simulink model "rotpen_quick_start"  (Simulink 7.9)
settings: Solver=ode1  StartTime=0.0  StopTime=inf  FixedStep=0.002  RelTol=1e-3
PostLoadFcn:
  | qc_set_target_type(getConfigSet(bdroot, 'QUARC Default Target Configuration'));
undefined symbols (not defined in the file): HIL, qc_get_step_size
libraries: quarc_library x3, simulink_extras x2, simulink x1
settings Model: Creator=Rchan  LastModifiedBy=User  SimulationMode=external  ExtModeTrigDuration=10000  ExtModeTrigDurationFloating=10000
settings SolverCC: PositivePriorityOrder=on
settings OptimizationCC: InitFltsAndDblsToZero=on
settings DebuggingCC: SaveWithParameterizedLinksMsg=none  MultiTaskDSMMsg=warning  MultiTaskCondExecSysMsg=none  FcnCallInpInsideContextMsg=Use local settings  StrictBusMsg=None
settings RTWCC: SystemTargetFile=quarc_win64.tlc  TemplateMakefile=quarc_default_tmf  Description=QUARC Win64 Target  ProcessScript=quarc_win64_make_rtw_hook
settings STFCustomTargetCC: TargetPreCompLibLocation=C:\PROGRA~3\QUARC\lib\2012a\win64\release  CodeReplacementLibrary=ANSI_C  GeneratePreprocessorConditionals=Disable all  SystemTargetFile=quarc_win64.tlc
settings GRTTargetCC: TargetPreCompLibLocation=C:\PROGRA~3\QUARC\lib\2012a\win64\release  ParMdlRefBuildCompliant=off  CompOptLevelCompliant=off  ConcurrentExecutionCompliant=off  CombineOutputUpdateFcns=off  MatFileLogging=off  GRTInterface=on  ExtMode=on  ExtModeMexFile=quarc_comm

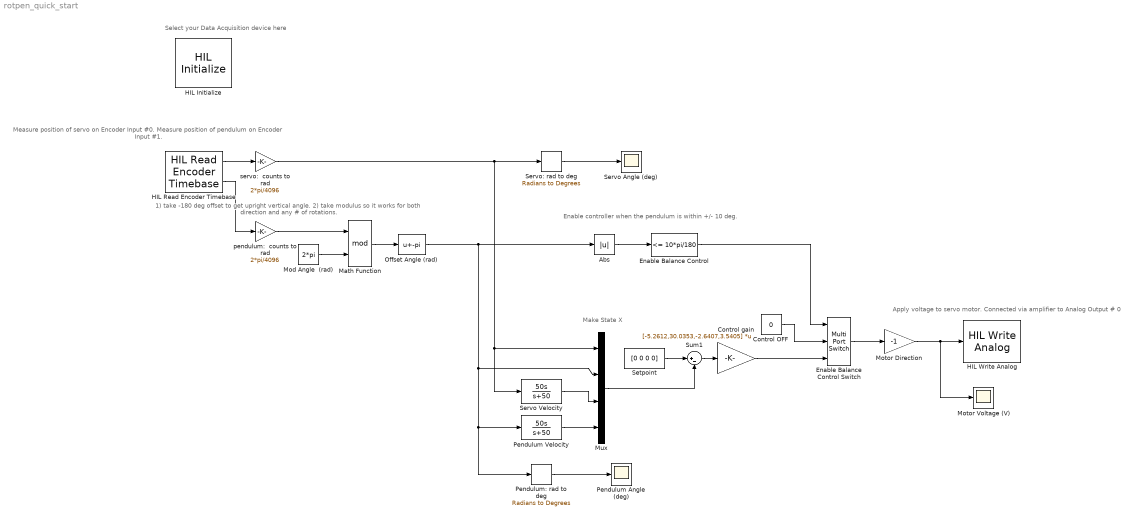
== system rotpen_quick_start ==
  note: Select your Data Acquisition device here
  note: Measure position of servo on Encoder Input #0.
      | Measure position of pendulum on Encoder Input #1.
  note: Apply voltage to servo motor.
      | Connected via amplifier to Analog Output # 0
  note: Enable controller when the
      | pendulum is within +/- 10 deg.
  note: 1) take -180 deg offset to get upright vertical angle.
      | 2) take modulus so it works for both direction
      | and any # of rotations.
  note: Make State X
  Abs : Abs
  Control OFF : Constant  Value=0
  Control gain : Gain  Gain=[-5.2612,30.0353,-2.6407,3.5405]  Multiplication=Matrix(K*u)
  Enable Balance Control : simulink/Logic and Bit Operations/Compare To Constant  relop=<=  const=10*pi/180  OutDataTypeStr=uint8  ZeroCross=off
  Enable Balance Control Switch : MultiPortSwitch  DataPortOrder=Zero-based contiguous  Inputs=2  zeroidx=on
  HIL Initialize : quarc_library/Data Acquisition/Generic/Configuration/HIL Initialize  Priority=-99  object_name=HIL-1  board_type=q8_usb  board_number=0  board_options=update_rate=normal;decimation=1  exclusive=off  active=off  hardware_clocks=[0:2]  clock_modes=[]  initial_clock_frequencies=[]  set_clock_params_at_start=off  set_clock_params_at_switch_in=off  set_clock_frequencies_at_start=off  set_clock_frequencies_at_switch_in=off  analog_input_channels=[0:7]  analog_input_maximums=10  analog_input_minimums=-10  set_analog_input_params_at_start=on  set_analog_input_params_at_switch_in=off  analog_output_channels=[0:7]  analog_output_maximums=10  analog_output_minimums=-10  initial_analog_outputs=[0]  final_analog_outputs=[0]  watchdog_analog_outputs=0  set_analog_output_params_at_start=on  set_analog_output_params_at_switch_in=off  set_analog_outputs_at_start=on  set_analog_outputs_at_switch_in=off  set_analog_outputs_at_terminate=on  set_analog_outputs_at_switch_out=off  set_analog_outputs_on_watchdog=off  digital_input_channels=[]  digital_output_channels=[]  digital_output_configuration=[]  initial_digital_outputs=[1]  final_digital_outputs=[1]  watchdog_digital_outputs=[1]  set_digital_output_params_at_start=off  set_digital_output_params_at_switch_in=off  set_digital_outputs_at_start=on  set_digital_outputs_at_switch_in=off  set_digital_outputs_at_terminate=on  set_digital_outputs_at_switch_out=off  set_digital_outputs_on_watchdog=off  encoder_channels=[0:7]  quadrature=[4]  encoder_filter_frequency=[]  initial_encoder_counts=[0]  set_encoder_params_at_start=on  set_encoder_params_at_switch_in=off  set_encoder_counts_at_start=on  set_encoder_counts_at_switch_in=off  pwm_channels=[0:7]  pwm_modes=0  pwm_frequency=99.532799999999995e6/4095  pwm_configuration=[0]  pwm_alignment=[0]  pwm_polarity=[1]  pwm_leading_deadband=[0]  pwm_trailing_deadband=[0]  initial_pwm_outputs=[0]  final_pwm_outputs=[0]  watchdog_pwm_outputs=[0]  set_pwm_params_at_start=on  set_pwm_params_at_switch_in=off  set_pwm_outputs_at_start=on  set_pwm_outputs_at_switch_in=off  set_pwm_outputs_at_terminate=on  set_pwm_outputs_at_switch_out=off  set_pwm_outputs_on_watchdog=off  other_output_channels=[]  initial_other_outputs=[]  final_other_outputs=[]  watchdog_other_outputs=[]  set_other_outputs_at_start=off  set_other_outputs_at_switch_in=off  set_other_outputs_at_terminate=off  set_other_outputs_at_switch_out=off  set_other_outputs_on_watchdog=off
  HIL Read Encoder Timebase : quarc_library/Data Acquisition/Generic/Timebases/HIL Read Encoder Timebase  object_name=HIL-1  clock=0  channels=0:1  samples_in_buffer=max(ceil(1/qc_get_step_size), 1)  active=on  vector_output=off  data_type_mode=Inherit via back propagation  data_type=double
  HIL Write Analog : quarc_library/Data Acquisition/Generic/Immediate I//O/HIL Write Analog  object_name=HIL-1  channels=0  sample_time=-1  active=off  vector_input=off
  Math Function : Math  Operator=mod  SaturateOnIntegerOverflow=on
  Mod Angle  (rad) : Constant  Value=2*pi
  "Motor Direction " : Gain  Gain=-1  SaturateOnIntegerOverflow=on  OutDataTypeStr=Inherit: Same as input  ParamDataTypeStr=Inherit: Same as input
  Motor Voltage (V) : Scope
      settings: TimeRange=10  YMin=-10  YMax=10
  Mux : Mux
  Offset Angle (rad) : Bias  Bias=-pi
  Pendulum Angle (deg) : Scope
      settings: YMin=-200  YMax=200  SaveName=ScopeData2
  Pendulum Velocity : TransferFcn  Numerator=[50 0]  Denominator=[1 50]
  Pendulum: rad to deg : simulink_extras/Transformations/Radians to Degrees
  Servo Angle (deg) : Scope
      settings: TimeRange=10  YMin=-40  YMax=40
  Servo Velocity : TransferFcn  Numerator=[50 0]  Denominator=[1 50]
  Servo: rad to deg : simulink_extras/Transformations/Radians to Degrees
  Setpoint : Constant  Value=[0 0 0 0]
  Sum1 : Sum  Inputs=|+-
  pendulum:  counts to rad : Gain  Gain=2*pi/4096
  servo:  counts to rad : Gain  Gain=2*pi/4096
  wires:
  HIL Read Encoder Timebase/1 -> servo:  counts to rad/1
  HIL Read Encoder Timebase/2 -> pendulum:  counts to rad/1
  Pendulum Velocity/1 -> Mux/4
  Mod Angle  (rad)/1 -> Math Function/2
  Math Function/1 -> Offset Angle (rad)/1
  Abs/1 -> Enable Balance Control/1
  Enable Balance Control/1 -> Enable Balance Control Switch/1
  Control OFF/1 -> Enable Balance Control Switch/2
  Sum1/1 -> Control gain/1
  Enable Balance Control Switch/1 -> "Motor Direction "/1
  Servo Velocity/1 -> Mux/3
  Servo: rad to deg/1 -> Servo Angle (deg)/1
  Pendulum: rad to deg/1 -> Pendulum Angle (deg)/1
  pendulum:  counts to rad/1 -> Math Function/1
  Setpoint/1 -> Sum1/1
  servo:  counts to rad/1 -> Servo: rad to deg/1, Mux/1, Servo Velocity/1
  Offset Angle (rad)/1 -> Mux/2, Pendulum Velocity/1, Pendulum: rad to deg/1, Abs/1
  Mux/1 -> Sum1/2
  Control gain/1 -> Enable Balance Control Switch/3
  "Motor Direction "/1 -> HIL Write Analog/1, Motor Voltage (V)/1
